simulink library "halin"  (R2021b)
settings: Solver=VariableStepAuto  StartTime=0.0  StopTime=10.0  RelTol=1e-3
undefined symbols (not defined in the file): KHAL_CAN1ABM1E2E_flg, KHAL_CAN1EPB1E2E_flg, KHAL_CAN1EPS1E2E_flg, KHAL_CAN1ESC1E2E_flg, KHAL_CAN1ESC5E2E_flg, KHAL_CAN3BMS1E2E_flg, KHAL_CAN3BMS6E2E_flg, KHAL_CAN3CCU1E2E_flg, KHAL_CAN3CCU2E2E_flg, KHAL_CAN3MCUNF1E2E_flg, KHAL_CAN3MCUNR1E2E_flg, KHAL_CAN3Shifter1E2E_flg, KHAL_CAN3Shifter2E2E_flg, KHAL_CAN6FCM2E2E_flg, KHAL_CAN6FCM4E2E_flg, TRUE
libraries: simulink x645, FVT_lib x207, hcu_lib x59
(part 8 of 23)

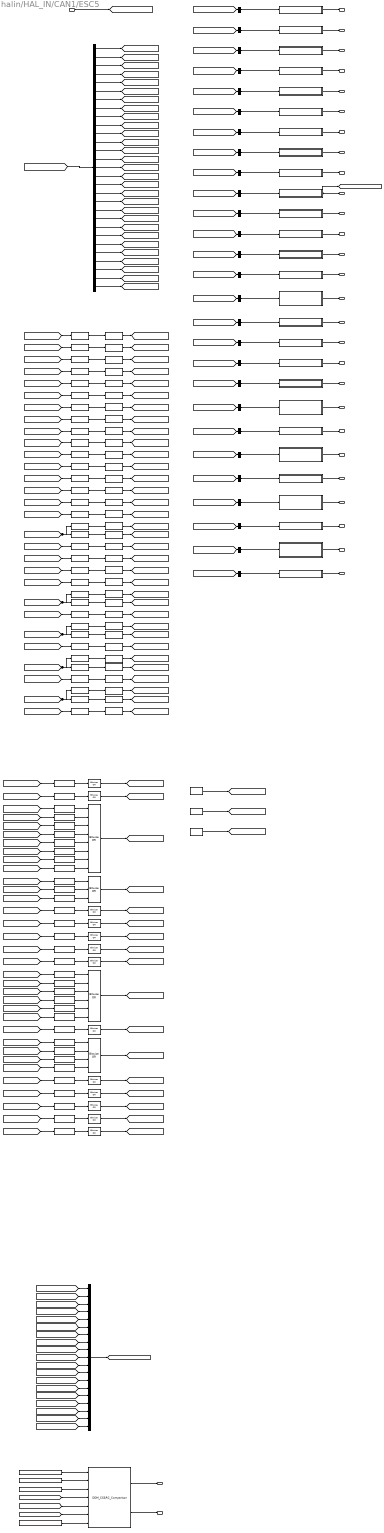
== system halin/HAL_IN/CAN1/ESC5 ==
  DT_CAN1_SG_ESC5 : Inport
  0x59 : Constant  Value=0x59
  0x6E : Constant  Value=0x6E
  ACCAvail : Subsystem
  AEBAvail : Subsystem
  ActBrkLampSta : Subsystem
  BitwiseAND{,1..33} (34 alike) : simulink/Logic and Bit Operations/Bitwise Operator  logicop=AND  UseBitMask=on  BitMask=0xFF  BitMaskRealWorld=Stored Integer
  BitwiseOR{,1,4..8,10,12..16} (13 alike) : simulink/Logic and Bit Operations/Bitwise Operator  logicop=OR  UseBitMask=off  BitMask=bin2dec('11011001')  BitMaskRealWorld=Stored Integer
  BitwiseOR11 : simulink/Logic and Bit Operations/Bitwise Operator  logicop=OR  UseBitMask=off  NumInputPorts=4  BitMask=bin2dec('11011001')  BitMaskRealWorld=Stored Integer
  BitwiseOR2 : simulink/Logic and Bit Operations/Bitwise Operator  logicop=OR  UseBitMask=off  NumInputPorts=8  BitMask=bin2dec('11011001')  BitMaskRealWorld=Stored Integer
  BitwiseOR3 : simulink/Logic and Bit Operations/Bitwise Operator  logicop=OR  UseBitMask=off  NumInputPorts=3  BitMask=bin2dec('11011001')  BitMaskRealWorld=Stored Integer
  BitwiseOR9 : simulink/Logic and Bit Operations/Bitwise Operator  logicop=OR  UseBitMask=off  NumInputPorts=6  BitMask=bin2dec('11011001')  BitMaskRealWorld=Stored Integer
  BrkDiscTempSta : Subsystem
  BrkPedalPos : Subsystem
  BrkPedalPosSta : Subsystem
  BrkSwSta : Subsystem
  BrkSwV : Subsystem
  DDM_CS&RC_Comparison : FVT_lib/hal/DDM_CS&RC_Comparison  MsgCycleTime=10
  Data Type Conversion{,1..33} (34 alike) : DataTypeConversion  OutDataTypeStr=uint8
  ESC5CS : Subsystem
  ESC5RC : Subsystem
  ESCADASSta : Subsystem
  ESCAPSSta : Subsystem
  ESCStandstill : Subsystem
  FrRBCActive : Subsystem
  FrntAxlTrqReqBrk : Subsystem
  KHAL_CAN1ESC5E2E_flg : Constant  Value=KHAL_CAN1ESC5E2E_flg
  LatAccel : Subsystem
  LatAccelV : Subsystem
  LeftShift : ArithShift  BitShiftNumber=1  BitShiftDirection=Left
  LeftShift1 : ArithShift  BitShiftNumber=3  BitShiftDirection=Left
  LeftShift{3..4,9..10,14..16,18} (8 alike) : ArithShift  BitShiftDirection=Left
  LeftShift11 : ArithShift  BitShiftNumber=4  BitShiftDirection=Left
  LeftShift12 : ArithShift  BitShiftNumber=5  BitShiftDirection=Left
  LeftShift13 : ArithShift  BitShiftNumber=7  BitShiftDirection=Left
  LeftShift17 : ArithShift  BitShiftNumber=3  BitShiftDirection=Left
  LeftShift19 : ArithShift  BitShiftNumber=4  BitShiftDirection=Left
  LeftShift2 : ArithShift  BitShiftNumber=2  BitShiftDirection=Left
  LeftShift20 : ArithShift  BitShiftNumber=5  BitShiftDirection=Left
  LeftShift21 : ArithShift  BitShiftNumber=2  BitShiftDirection=Left
  LeftShift22 : ArithShift  BitShiftNumber=1  BitShiftDirection=Left
  LeftShift23 : ArithShift  BitShiftNumber=2  BitShiftDirection=Left
  LeftShift5 : ArithShift  BitShiftNumber=4  BitShiftDirection=Left
  LeftShift6 : ArithShift  BitShiftNumber=6  BitShiftDirection=Left
  LeftShift7 : ArithShift  BitShiftNumber=7  BitShiftDirection=Left
  LeftShift8 : ArithShift  BitShiftNumber=1  BitShiftDirection=Left
  LongAccel : Subsystem
  LongAccelV : Subsystem
  MCPressure : Subsystem
  MCPressureV : Subsystem
  MessageRollingCounter : FVT_lib/hal/MessageRollingCounter  CounterMAX=14  task_time_ms=5  msg_time_ms=10
  MeterIndVehSpeed : Subsystem
  Mux : Mux  Inputs=19
  RDCActive : Subsystem
  RearAxlTrqReqBrk : Subsystem
  RightShift{,2,6,8} (4 alike) : ArithShift  BitShiftNumber=8
  RightShift{1,3,7,9} (4 alike) : ArithShift
  RightShift4 : ArithShift  BitShiftNumber=4
  RightShift5 : ArithShift  BitShiftNumber=-4
  RrRBCActive : Subsystem
  YawRate : Subsystem
  YawRateV : Subsystem
  bus_selector : BusSelector  OutputSignals=CAN1_ACCAvail,CAN1_AEBAvail,CAN1_ActBrkLamp_Sta,CAN1_BrkDiscTempSta,CAN1_BrkPedalPos,CAN1_BrkPedalPos_Sta,CAN1_BrkSw_Sta,CAN1_BrkSw_V,CAN1_DecErrSta,CAN1_ESC5_CS,CAN1_ESC5_RC,CAN1_ESC_ADAS_Sta,CAN1_ESC_APS_Sta,CAN1_ESC_DriverBrkOverride,CAN1_ESC_Standstill,CAN1_Fr_RBC_Active,CAN1_FrntAxlTrqReq_Brk,CAN1_LatAccel,CAN1_LatAccel_V,CAN1_LongAccel,CAN1_LongAccel_V,CAN1_MCPressure,CAN1_MCPressure_V,CAN1_Meter_Ind_VehSpeed,CAN1_RDC_Active,CAN1_RearAxlTrqReq_Brk,CAN1_Rr_RBC_Active,CAN1_YawRate,CAN1_YawRate_V
  bus_selector1 : BusSelector  OutputSignals=CAN1_ACCAvail
  bus_selector10 : BusSelector  OutputSignals=CAN1_ESC5_RC
  bus_selector11 : BusSelector  OutputSignals=CAN1_ESC_ADAS_Sta
  bus_selector12 : BusSelector  OutputSignals=CAN1_ESC_APS_Sta
  bus_selector13 : BusSelector  OutputSignals=CAN1_ESC_Standstill
  bus_selector14 : BusSelector  OutputSignals=CAN1_Fr_RBC_Active
  bus_selector15 : BusSelector  OutputSignals=CAN1_FrntAxlTrqReq_Brk
  bus_selector16 : BusSelector  OutputSignals=CAN1_LatAccel
  bus_selector17 : BusSelector  OutputSignals=CAN1_LatAccel_V
  bus_selector18 : BusSelector  OutputSignals=CAN1_LongAccel
  bus_selector19 : BusSelector  OutputSignals=CAN1_LongAccel_V
  bus_selector2 : BusSelector  OutputSignals=CAN1_AEBAvail
  bus_selector20 : BusSelector  OutputSignals=CAN1_MCPressure
  bus_selector21 : BusSelector  OutputSignals=CAN1_MCPressure_V
  bus_selector22 : BusSelector  OutputSignals=CAN1_Meter_Ind_VehSpeed
  bus_selector23 : BusSelector  OutputSignals=CAN1_RDC_Active
  bus_selector24 : BusSelector  OutputSignals=CAN1_RearAxlTrqReq_Brk
  bus_selector25 : BusSelector  OutputSignals=CAN1_Rr_RBC_Active
  bus_selector26 : BusSelector  OutputSignals=CAN1_YawRate
  bus_selector27 : BusSelector  OutputSignals=CAN1_YawRate_V
  bus_selector3 : BusSelector  OutputSignals=CAN1_ActBrkLamp_Sta
  bus_selector4 : BusSelector  OutputSignals=CAN1_BrkDiscTempSta
  bus_selector5 : BusSelector  OutputSignals=CAN1_BrkPedalPos
  bus_selector6 : BusSelector  OutputSignals=CAN1_BrkPedalPos_Sta
  bus_selector7 : BusSelector  OutputSignals=CAN1_BrkSw_Sta
  bus_selector8 : BusSelector  OutputSignals=CAN1_BrkSw_V
  bus_selector9 : BusSelector  OutputSignals=CAN1_ESC5_CS
  constant : Constant  Value=0x0  OutDataTypeStr=uint8
  constant1 : Constant  Value=0x0  OutDataTypeStr=uint8
  constant2 : Constant  Value=0x0  OutDataTypeStr=uint8
  VHAL_ESC5CSErr_flg : Outport
  VHAL_ESC5RCErr_flg : Outport  Port=2
  VHAL_ACCAvail_flg : Outport  Port=3
  VHAL_AEBAvail_flg : Outport  Port=4
  VHAL_ActBrkLampSta_flg : Outport  Port=5
  VHAL_BrkDiscTempSta_flg : Outport  Port=6
  VHAL_BrkPedalPos_pct : Outport  Port=7
  VHAL_BrkPedalPosSta_flg : Outport  Port=8
  VHAL_BrkSwSta_flg : Outport  Port=9
  VHAL_BrkSwV_flg : Outport  Port=10
  VHAL_ESC5CS_enum : Outport  Port=11
  VHAL_ESC5RC_enum : Outport  Port=12
  VHAL_ESCADASSta_enum : Outport  Port=13
  VHAL_ESCAPSSta_enum : Outport  Port=14
  VHAL_ESCStandstill_flg : Outport  Port=15
  VHAL_FrRBCActive_flg : Outport  Port=16
  VHAL_FrntAxlTrqReqBrk_Nm : Outport  Port=17
  VHAL_LatAccel_Gps : Outport  Port=18
  VHAL_LatAccelV_flg : Outport  Port=19
  VHAL_LongAccel_Gps : Outport  Port=20
  VHAL_LongAccelV_flg : Outport  Port=21
  VHAL_MCPressure_bar : Outport  Port=22
  VHAL_MCPressureV_flg : Outport  Port=23
  VHAL_MeterIndVehSpeed_kph : Outport  Port=24
  VHAL_RDCActive_enum : Outport  Port=25
  VHAL_RearAxlTrqReqBrk_Nm : Outport  Port=26
  VHAL_RrRBCActive_flg : Outport  Port=27
  VHAL_YawRate_degps : Outport  Port=28
  VHAL_YawRateV_flg : Outport  Port=29
  wires:
  DT_CAN1_SG_ESC5/1 -> [DT_CAN1_SG_ESC5]
  [DT_CAN1_SG_ESC5] -> bus_selector/1
  bus_selector/1 -> [CAN1_ACCAvail]  "<CAN1_ACCAvail>"
  [CAN1_ACCAvail] -> LeftShift/1
  LeftShift/1 -> BitwiseAND/1
  BitwiseAND/1 -> [Byte_2_CAN1_ACCAvail]
  bus_selector/2 -> [CAN1_AEBAvail]  "<CAN1_AEBAvail>"
  [CAN1_AEBAvail] -> LeftShift1/1
  LeftShift1/1 -> BitwiseAND1/1
  BitwiseAND1/1 -> [Byte_9_CAN1_AEBAvail]
  bus_selector/3 -> [CAN1_ActBrkLamp_Sta]  "<CAN1_ActBrkLamp_Sta>"
  [CAN1_ActBrkLamp_Sta] -> LeftShift2/1
  LeftShift2/1 -> BitwiseAND2/1
  BitwiseAND2/1 -> [Byte_9_CAN1_ActBrkLamp_Sta]
  bus_selector/4 -> [CAN1_BrkDiscTempSta]  "<CAN1_BrkDiscTempSta>"
  [CAN1_BrkDiscTempSta] -> LeftShift3/1
  LeftShift3/1 -> BitwiseAND3/1
  BitwiseAND3/1 -> [Byte_2_CAN1_BrkDiscTempSta]
  bus_selector/5 -> [CAN1_BrkPedalPos]  "<CAN1_BrkPedalPos>"
  [CAN1_BrkPedalPos] -> LeftShift4/1
  LeftShift4/1 -> BitwiseAND4/1
  BitwiseAND4/1 -> [Byte_12_CAN1_BrkPedalPos]
  bus_selector/6 -> [CAN1_BrkPedalPos_Sta]  "<CAN1_BrkPedalPos_Sta>"
  [CAN1_BrkPedalPos_Sta] -> LeftShift5/1
  LeftShift5/1 -> BitwiseAND5/1
  BitwiseAND5/1 -> [Byte_9_CAN1_BrkPedalPos_Sta]
  bus_selector/7 -> [CAN1_BrkSw_Sta]  "<CAN1_BrkSw_Sta>"
  [CAN1_BrkSw_Sta] -> LeftShift6/1
  LeftShift6/1 -> BitwiseAND6/1
  BitwiseAND6/1 -> [Byte_2_CAN1_BrkSw_Sta]
  bus_selector/8 -> [CAN1_BrkSw_V]  "<CAN1_BrkSw_V>"
  [CAN1_BrkSw_V] -> LeftShift7/1
  LeftShift7/1 -> BitwiseAND7/1
  BitwiseAND7/1 -> [Byte_2_CAN1_BrkSw_V]
  bus_selector/9 -> [CAN1_DecErrSta]  "<CAN1_DecErrSta>"
  [CAN1_DecErrSta] -> LeftShift8/1
  LeftShift8/1 -> BitwiseAND8/1
  BitwiseAND8/1 -> [Byte_9_CAN1_DecErrSta]
  bus_selector/10 -> [CAN1_ESC5_CS]  "<CAN1_ESC5_CS>"
  [CAN1_ESC5_CS] -> LeftShift9/1
  LeftShift9/1 -> BitwiseAND9/1
  BitwiseAND9/1 -> [Byte_0_CAN1_ESC5_CS]
  bus_selector/11 -> [CAN1_ESC5_RC]  "<CAN1_ESC5_RC>"
  [CAN1_ESC5_RC] -> LeftShift10/1
  LeftShift10/1 -> BitwiseAND10/1
  BitwiseAND10/1 -> [Byte_1_CAN1_ESC5_RC]
  bus_selector/12 -> [CAN1_ESC_ADAS_Sta]  "<CAN1_ESC_ADAS_Sta>"
  [CAN1_ESC_ADAS_Sta] -> LeftShift11/1
  LeftShift11/1 -> BitwiseAND11/1
  BitwiseAND11/1 -> [Byte_3_CAN1_ESC_ADAS_Sta]
  bus_selector/13 -> [CAN1_ESC_APS_Sta]  "<CAN1_ESC_APS_Sta>"
  [CAN1_ESC_APS_Sta] -> LeftShift12/1
  LeftShift12/1 -> BitwiseAND12/1
  BitwiseAND12/1 -> [Byte_9_CAN1_ESC_APS_Sta]
  bus_selector/14 -> [CAN1_ESC_DriverBrkOverride]  "<CAN1_ESC_DriverBrkOverride>"
  [CAN1_ESC_DriverBrkOverride] -> LeftShift13/1
  LeftShift13/1 -> BitwiseAND13/1
  BitwiseAND13/1 -> [Byte_3_CAN1_ESC_DriverBrkOverride]
  bus_selector/15 -> [CAN1_ESC_Standstill]  "<CAN1_ESC_Standstill>"
  [CAN1_ESC_Standstill] -> LeftShift14/1
  LeftShift14/1 -> BitwiseAND14/1
  BitwiseAND14/1 -> [Byte_9_CAN1_ESC_Standstill]
  bus_selector/16 -> [CAN1_Fr_RBC_Active]  "<CAN1_Fr_RBC_Active>"
  [CAN1_Fr_RBC_Active] -> LeftShift15/1
  LeftShift15/1 -> BitwiseAND15/1
  BitwiseAND15/1 -> [Byte_11_CAN1_Fr_RBC_Active]
  bus_selector/17 -> [CAN1_FrntAxlTrqReq_Brk]  "<CAN1_FrntAxlTrqReq_Brk>"
  [CAN1_FrntAxlTrqReq_Brk] -> RightShift/1, RightShift1/1
  RightShift/1 -> BitwiseAND16/1
  BitwiseAND16/1 -> [Byte_15_CAN1_FrntAxlTrqReq_Brk]
  RightShift1/1 -> BitwiseAND17/1
  BitwiseAND17/1 -> [Byte_16_CAN1_FrntAxlTrqReq_Brk]
  bus_selector/18 -> [CAN1_LatAccel]  "<CAN1_LatAccel>"
  [CAN1_LatAccel] -> LeftShift16/1
  LeftShift16/1 -> BitwiseAND18/1
  BitwiseAND18/1 -> [Byte_6_CAN1_LatAccel]
  bus_selector/19 -> [CAN1_LatAccel_V]  "<CAN1_LatAccel_V>"
  [CAN1_LatAccel_V] -> LeftShift17/1
  LeftShift17/1 -> BitwiseAND19/1
  BitwiseAND19/1 -> [Byte_2_CAN1_LatAccel_V]
  bus_selector/20 -> [CAN1_LongAccel]  "<CAN1_LongAccel>"
  [CAN1_LongAccel] -> LeftShift18/1
  LeftShift18/1 -> BitwiseAND20/1
  BitwiseAND20/1 -> [Byte_5_CAN1_LongAccel]
  bus_selector/21 -> [CAN1_LongAccel_V]  "<CAN1_LongAccel_V>"
  [CAN1_LongAccel_V] -> LeftShift19/1
  LeftShift19/1 -> BitwiseAND21/1
  BitwiseAND21/1 -> [Byte_2_CAN1_LongAccel_V]
  bus_selector/22 -> [CAN1_MCPressure]  "<CAN1_MCPressure>"
  [CAN1_MCPressure] -> RightShift2/1, RightShift3/1
  RightShift2/1 -> BitwiseAND22/1
  BitwiseAND22/1 -> [Byte_3_CAN1_MCPressure]
  RightShift3/1 -> BitwiseAND23/1
  BitwiseAND23/1 -> [Byte_4_CAN1_MCPressure]
  bus_selector/23 -> [CAN1_MCPressure_V]  "<CAN1_MCPressure_V>"
  [CAN1_MCPressure_V] -> LeftShift20/1
  LeftShift20/1 -> BitwiseAND24/1
  BitwiseAND24/1 -> [Byte_2_CAN1_MCPressure_V]
  bus_selector/24 -> [CAN1_Meter_Ind_VehSpeed]  "<CAN1_Meter_Ind_VehSpeed>"
  [CAN1_Meter_Ind_VehSpeed] -> RightShift4/1, RightShift5/1
  RightShift4/1 -> BitwiseAND25/1
  BitwiseAND25/1 -> [Byte_10_CAN1_Meter_Ind_VehSpeed]
  RightShift5/1 -> BitwiseAND26/1
  BitwiseAND26/1 -> [Byte_11_CAN1_Meter_Ind_VehSpeed]
  bus_selector/25 -> [CAN1_RDC_Active]  "<CAN1_RDC_Active>"
  [CAN1_RDC_Active] -> LeftShift21/1
  LeftShift21/1 -> BitwiseAND27/1
  BitwiseAND27/1 -> [Byte_11_CAN1_RDC_Active]
  bus_selector/26 -> [CAN1_RearAxlTrqReq_Brk]  "<CAN1_RearAxlTrqReq_Brk>"
  [CAN1_RearAxlTrqReq_Brk] -> RightShift6/1, RightShift7/1
  RightShift6/1 -> BitwiseAND28/1
  BitwiseAND28/1 -> [Byte_13_CAN1_RearAxlTrqReq_Brk]
  RightShift7/1 -> BitwiseAND29/1
  BitwiseAND29/1 -> [Byte_14_CAN1_RearAxlTrqReq_Brk]
  bus_selector/27 -> [CAN1_Rr_RBC_Active]  "<CAN1_Rr_RBC_Active>"
  [CAN1_Rr_RBC_Active] -> LeftShift22/1
  LeftShift22/1 -> BitwiseAND30/1
  BitwiseAND30/1 -> [Byte_11_CAN1_Rr_RBC_Active]
  bus_selector/28 -> [CAN1_YawRate]  "<CAN1_YawRate>"
  [CAN1_YawRate] -> RightShift8/1, RightShift9/1
  RightShift8/1 -> BitwiseAND31/1
  BitwiseAND31/1 -> [Byte_7_CAN1_YawRate]
  RightShift9/1 -> BitwiseAND32/1
  BitwiseAND32/1 -> [Byte_8_CAN1_YawRate]
  bus_selector/29 -> [CAN1_YawRate_V]  "<CAN1_YawRate_V>"
  [CAN1_YawRate_V] -> LeftShift23/1
  LeftShift23/1 -> BitwiseAND33/1
  BitwiseAND33/1 -> [Byte_2_CAN1_YawRate_V]
  Data Type Conversion/1 -> BitwiseOR/1
  [Byte_0_CAN1_ESC5_CS] -> Data Type Conversion/1
  BitwiseOR/1 -> [Byte_0]
  Data Type Conversion1/1 -> BitwiseOR1/1
  [Byte_1_CAN1_ESC5_RC] -> Data Type Conversion1/1
  BitwiseOR1/1 -> [Byte_1]
  Data Type Conversion2/1 -> BitwiseOR2/1
  [Byte_2_CAN1_ACCAvail] -> Data Type Conversion2/1
  Data Type Conversion3/1 -> BitwiseOR2/2
  [Byte_2_CAN1_BrkDiscTempSta] -> Data Type Conversion3/1
  Data Type Conversion4/1 -> BitwiseOR2/3
  [Byte_2_CAN1_BrkSw_Sta] -> Data Type Conversion4/1
  Data Type Conversion5/1 -> BitwiseOR2/4
  [Byte_2_CAN1_BrkSw_V] -> Data Type Conversion5/1
  Data Type Conversion6/1 -> BitwiseOR2/5
  [Byte_2_CAN1_LatAccel_V] -> Data Type Conversion6/1
  Data Type Conversion7/1 -> BitwiseOR2/6
  [Byte_2_CAN1_LongAccel_V] -> Data Type Conversion7/1
  Data Type Conversion8/1 -> BitwiseOR2/7
  [Byte_2_CAN1_MCPressure_V] -> Data Type Conversion8/1
  Data Type Conversion9/1 -> BitwiseOR2/8
  [Byte_2_CAN1_YawRate_V] -> Data Type Conversion9/1
  BitwiseOR2/1 -> [Byte_2]
  Data Type Conversion10/1 -> BitwiseOR3/1
  [Byte_3_CAN1_ESC_ADAS_Sta] -> Data Type Conversion10/1
  Data Type Conversion11/1 -> BitwiseOR3/2
  [Byte_3_CAN1_ESC_DriverBrkOverride] -> Data Type Conversion11/1
  Data Type Conversion12/1 -> BitwiseOR3/3
  [Byte_3_CAN1_MCPressure] -> Data Type Conversion12/1
  BitwiseOR3/1 -> [Byte_3]
  Data Type Conversion13/1 -> BitwiseOR4/1
  [Byte_4_CAN1_MCPressure] -> Data Type Conversion13/1
  BitwiseOR4/1 -> [Byte_4]
  Data Type Conversion14/1 -> BitwiseOR5/1
  [Byte_5_CAN1_LongAccel] -> Data Type Conversion14/1
  BitwiseOR5/1 -> [Byte_5]
  Data Type Conversion15/1 -> BitwiseOR6/1
  [Byte_6_CAN1_LatAccel] -> Data Type Conversion15/1
  BitwiseOR6/1 -> [Byte_6]
  Data Type Conversion16/1 -> BitwiseOR7/1
  [Byte_7_CAN1_YawRate] -> Data Type Conversion16/1
  BitwiseOR7/1 -> [Byte_7]
  Data Type Conversion17/1 -> BitwiseOR8/1
  [Byte_8_CAN1_YawRate] -> Data Type Conversion17/1
  BitwiseOR8/1 -> [Byte_8]
  Data Type Conversion18/1 -> BitwiseOR9/1
  [Byte_9_CAN1_AEBAvail] -> Data Type Conversion18/1
  Data Type Conversion19/1 -> BitwiseOR9/2
  [Byte_9_CAN1_ActBrkLamp_Sta] -> Data Type Conversion19/1
  Data Type Conversion20/1 -> BitwiseOR9/3
  [Byte_9_CAN1_BrkPedalPos_Sta] -> Data Type Conversion20/1
  Data Type Conversion21/1 -> BitwiseOR9/4
  [Byte_9_CAN1_DecErrSta] -> Data Type Conversion21/1
  Data Type Conversion22/1 -> BitwiseOR9/5
  [Byte_9_CAN1_ESC_APS_Sta] -> Data Type Conversion22/1
  Data Type Conversion23/1 -> BitwiseOR9/6
  [Byte_9_CAN1_ESC_Standstill] -> Data Type Conversion23/1
  BitwiseOR9/1 -> [Byte_9]
  Data Type Conversion24/1 -> BitwiseOR10/1
  [Byte_10_CAN1_Meter_Ind_VehSpeed] -> Data Type Conversion24/1
  BitwiseOR10/1 -> [Byte_10]
  Data Type Conversion25/1 -> BitwiseOR11/1
  [Byte_11_CAN1_Fr_RBC_Active] -> Data Type Conversion25/1
  Data Type Conversion26/1 -> BitwiseOR11/2
  [Byte_11_CAN1_Meter_Ind_VehSpeed] -> Data Type Conversion26/1
  Data Type Conversion27/1 -> BitwiseOR11/3
  [Byte_11_CAN1_RDC_Active] -> Data Type Conversion27/1
  Data Type Conversion28/1 -> BitwiseOR11/4
  [Byte_11_CAN1_Rr_RBC_Active] -> Data Type Conversion28/1
  BitwiseOR11/1 -> [Byte_11]
  Data Type Conversion29/1 -> BitwiseOR12/1
  [Byte_12_CAN1_BrkPedalPos] -> Data Type Conversion29/1
  BitwiseOR12/1 -> [Byte_12]
  Data Type Conversion30/1 -> BitwiseOR13/1
  [Byte_13_CAN1_RearAxlTrqReq_Brk] -> Data Type Conversion30/1
  BitwiseOR13/1 -> [Byte_13]
  Data Type Conversion31/1 -> BitwiseOR14/1
  [Byte_14_CAN1_RearAxlTrqReq_Brk] -> Data Type Conversion31/1
  BitwiseOR14/1 -> [Byte_14]
  Data Type Conversion32/1 -> BitwiseOR15/1
  [Byte_15_CAN1_FrntAxlTrqReq_Brk] -> Data Type Conversion32/1
  BitwiseOR15/1 -> [Byte_15]
  Data Type Conversion33/1 -> BitwiseOR16/1
  [Byte_16_CAN1_FrntAxlTrqReq_Brk] -> Data Type Conversion33/1
  BitwiseOR16/1 -> [Byte_16]
  constant/1 -> [Byte_17]
  constant1/1 -> [Byte_18]
  constant2/1 -> [Byte_19]
  [Byte_1] -> Mux/1
  [Byte_2] -> Mux/2
  [Byte_3] -> Mux/3
  [Byte_4] -> Mux/4
  [Byte_5] -> Mux/5
  [Byte_6] -> Mux/6
  [Byte_7] -> Mux/7
  [Byte_8] -> Mux/8
  [Byte_9] -> Mux/9
  [Byte_10] -> Mux/10
  [Byte_11] -> Mux/11
  [Byte_12] -> Mux/12
  [Byte_13] -> Mux/13
  [Byte_14] -> Mux/14
  [Byte_15] -> Mux/15
  [Byte_16] -> Mux/16
  [Byte_17] -> Mux/17
  [Byte_18] -> Mux/18
  [Byte_19] -> Mux/19
  Mux/1 -> [VHAL_CAN1ESC5noCS_raw]
  KHAL_CAN1ESC5E2E_flg/1 -> DDM_CS&RC_Comparison/1
  0x59/1 -> DDM_CS&RC_Comparison/2
  0x6E/1 -> DDM_CS&RC_Comparison/3
  [VHAL_CAN1ESC5noCS_raw] -> DDM_CS&RC_Comparison/4
  [Byte_0] -> DDM_CS&RC_Comparison/5
  [RC_ECU] -> DDM_CS&RC_Comparison/6
  MessageRollingCounter/1 -> DDM_CS&RC_Comparison/7
  DDM_CS&RC_Comparison/1 -> VHAL_ESC5CSErr_flg/1
  DDM_CS&RC_Comparison/2 -> VHAL_ESC5RCErr_flg/1
  [DT_CAN1_SG_ESC5] -> bus_selector1/1
  bus_selector1/1 -> ACCAvail/1(ACCAvail)  "<CAN1_ACCAvail>"
  ACCAvail/1(VHAL_ACCAvail_flg) -> VHAL_ACCAvail_flg/1
  [DT_CAN1_SG_ESC5] -> bus_selector2/1
  bus_selector2/1 -> AEBAvail/1(AEBAvail)  "<CAN1_AEBAvail>"
  AEBAvail/1(VHAL_AEBAvail_flg) -> VHAL_AEBAvail_flg/1
  [DT_CAN1_SG_ESC5] -> bus_selector3/1
  bus_selector3/1 -> ActBrkLampSta/1(ActBrkLamp_Sta)  "<CAN1_ActBrkLamp_Sta>"
  ActBrkLampSta/1(VHAL_ActBrkLampSta_flg) -> VHAL_ActBrkLampSta_flg/1
  [DT_CAN1_SG_ESC5] -> bus_selector4/1
  bus_selector4/1 -> BrkDiscTempSta/1(BrkDiscTempSta)  "<CAN1_BrkDiscTempSta>"
  BrkDiscTempSta/1(VHAL_BrkDiscTempSta_flg) -> VHAL_BrkDiscTempSta_flg/1
  [DT_CAN1_SG_ESC5] -> bus_selector5/1
  bus_selector5/1 -> BrkPedalPos/1(BrkPedalPos)  "<CAN1_BrkPedalPos>"
  BrkPedalPos/1(VHAL_BrkPedalPos_pct) -> VHAL_BrkPedalPos_pct/1
  [DT_CAN1_SG_ESC5] -> bus_selector6/1
  bus_selector6/1 -> BrkPedalPosSta/1(BrkPedalPos_Sta)  "<CAN1_BrkPedalPos_Sta>"
  BrkPedalPosSta/1(VHAL_BrkPedalPosSta_flg) -> VHAL_BrkPedalPosSta_flg/1
  [DT_CAN1_SG_ESC5] -> bus_selector7/1
  bus_selector7/1 -> BrkSwSta/1(BrkSw_Sta)  "<CAN1_BrkSw_Sta>"
  BrkSwSta/1(VHAL_BrkSwSta_flg) -> VHAL_BrkSwSta_flg/1
  [DT_CAN1_SG_ESC5] -> bus_selector8/1
  bus_selector8/1 -> BrkSwV/1(BrkSw_V)  "<CAN1_BrkSw_V>"
  BrkSwV/1(VHAL_BrkSwV_flg) -> VHAL_BrkSwV_flg/1
  [DT_CAN1_SG_ESC5] -> bus_selector9/1
  bus_selector9/1 -> ESC5CS/1(ESC5_CS)  "<CAN1_ESC5_CS>"
  ESC5CS/1(VHAL_ESC5CS_enum) -> VHAL_ESC5CS_enum/1
  [DT_CAN1_SG_ESC5] -> bus_selector10/1
  bus_selector10/1 -> ESC5RC/1(ESC5_RC)  "<CAN1_ESC5_RC>"
  ESC5RC/1(VHAL_ESC5RC_enum) -> VHAL_ESC5RC_enum/1, [RC_ECU]
  [DT_CAN1_SG_ESC5] -> bus_selector11/1
  bus_selector11/1 -> ESCADASSta/1(ESC_ADAS_Sta)  "<CAN1_ESC_ADAS_Sta>"
  ESCADASSta/1(VHAL_ESCADASSta_enum) -> VHAL_ESCADASSta_enum/1
  [DT_CAN1_SG_ESC5] -> bus_selector12/1
  bus_selector12/1 -> ESCAPSSta/1(ESC_APS_Sta)  "<CAN1_ESC_APS_Sta>"
  ESCAPSSta/1(VHAL_ESCAPSSta_enum) -> VHAL_ESCAPSSta_enum/1
  [DT_CAN1_SG_ESC5] -> bus_selector13/1
  bus_selector13/1 -> ESCStandstill/1(ESC_Standstill)  "<CAN1_ESC_Standstill>"
  ESCStandstill/1(VHAL_ESCStandstill_flg) -> VHAL_ESCStandstill_flg/1
  [DT_CAN1_SG_ESC5] -> bus_selector14/1
  bus_selector14/1 -> FrRBCActive/1(Fr_RBC_Active)  "<CAN1_Fr_RBC_Active>"
  FrRBCActive/1(VHAL_FrRBCActive_flg) -> VHAL_FrRBCActive_flg/1
  [DT_CAN1_SG_ESC5] -> bus_selector15/1
  bus_selector15/1 -> FrntAxlTrqReqBrk/1(FrntAxlTrqReq_Brk)  "<CAN1_FrntAxlTrqReq_Brk>"
  FrntAxlTrqReqBrk/1(VHAL_FrntAxlTrqReqBrk_Nm) -> VHAL_FrntAxlTrqReqBrk_Nm/1
  [DT_CAN1_SG_ESC5] -> bus_selector16/1
  bus_selector16/1 -> LatAccel/1(LatAccel)  "<CAN1_LatAccel>"
  LatAccel/1(VHAL_LatAccel_Gps) -> VHAL_LatAccel_Gps/1
  [DT_CAN1_SG_ESC5] -> bus_selector17/1
  bus_selector17/1 -> LatAccelV/1(LatAccel_V)  "<CAN1_LatAccel_V>"
  LatAccelV/1(VHAL_LatAccelV_flg) -> VHAL_LatAccelV_flg/1
  [DT_CAN1_SG_ESC5] -> bus_selector18/1
  bus_selector18/1 -> LongAccel/1(LongAccel)  "<CAN1_LongAccel>"
  LongAccel/1(VHAL_LongAccel_Gps) -> VHAL_LongAccel_Gps/1
  [DT_CAN1_SG_ESC5] -> bus_selector19/1
  bus_selector19/1 -> LongAccelV/1(LongAccel_V)  "<CAN1_LongAccel_V>"
  LongAccelV/1(VHAL_LongAccelV_flg) -> VHAL_LongAccelV_flg/1
  [DT_CAN1_SG_ESC5] -> bus_selector20/1
  bus_selector20/1 -> MCPressure/1(MCPressure)  "<CAN1_MCPressure>"
  MCPressure/1(VHAL_MCPressure_bar) -> VHAL_MCPressure_bar/1
  [DT_CAN1_SG_ESC5] -> bus_selector21/1
  bus_selector21/1 -> MCPressureV/1(MCPressure_V)  "<CAN1_MCPressure_V>"
  MCPressureV/1(VHAL_MCPressureV_flg) -> VHAL_MCPressureV_flg/1
  [DT_CAN1_SG_ESC5] -> bus_selector22/1
  bus_selector22/1 -> MeterIndVehSpeed/1(Meter_Ind_VehSpeed)  "<CAN1_Meter_Ind_VehSpeed>"
  MeterIndVehSpeed/1(VHAL_MeterIndVehSpeed_kph) -> VHAL_MeterIndVehSpeed_kph/1
  [DT_CAN1_SG_ESC5] -> bus_selector23/1
  bus_selector23/1 -> RDCActive/1(RDC_Active)  "<CAN1_RDC_Active>"
  RDCActive/1(VHAL_RDCActive_enum) -> VHAL_RDCActive_enum/1
  [DT_CAN1_SG_ESC5] -> bus_selector24/1
  bus_selector24/1 -> RearAxlTrqReqBrk/1(RearAxlTrqReq_Brk)  "<CAN1_RearAxlTrqReq_Brk>"
  RearAxlTrqReqBrk/1(VHAL_RearAxlTrqReqBrk_Nm) -> VHAL_RearAxlTrqReqBrk_Nm/1
  [DT_CAN1_SG_ESC5] -> bus_selector25/1
  bus_selector25/1 -> RrRBCActive/1(Rr_RBC_Active)  "<CAN1_Rr_RBC_Active>"
  RrRBCActive/1(VHAL_RrRBCActive_flg) -> VHAL_RrRBCActive_flg/1
  [DT_CAN1_SG_ESC5] -> bus_selector26/1
  bus_selector26/1 -> YawRate/1(YawRate)  "<CAN1_YawRate>"
  YawRate/1(VHAL_YawRate_degps) -> VHAL_YawRate_degps/1
  [DT_CAN1_SG_ESC5] -> bus_selector27/1
  bus_selector27/1 -> YawRateV/1(YawRate_V)  "<CAN1_YawRate_V>"
  YawRateV/1(VHAL_YawRateV_flg) -> VHAL_YawRateV_flg/1

== system halin/HAL_IN/CAN1/VHAL_CANMsgInvalidABM1_flg ==
  Cast To Boolean13 : DataTypeConversion  OutDataTypeStr=boolean
  Constant : Constant  Value=TRUE
  Latch13 : hcu_lib/Basic_Blocks/Latch
  Switch13 : Switch  Criteria=u2 ~= 0
  Unit Delay : UnitDelay  SampleTime=-1  HasFrameUpgradeWarning=on
  UnitConverter : DataTypeConversion  OutDataTypeStr=boolean
  Out : Outport
  wires:
  Constant/1 -> Switch13/3
  Unit Delay/1 -> Cast To Boolean13/1
  Cast To Boolean13/1 -> Switch13/1, Latch13/1
  Switch13/1 -> UnitConverter/1
  Latch13/1 -> Switch13/2
  UnitConverter/1 -> Unit Delay/1, Out/1  "VHAL_CANMsgInvalidABM1_flg"

== system halin/HAL_IN/CAN1/VHAL_CANMsgInvalidEPB1_flg ==
  Cast To Boolean13 : DataTypeConversion  OutDataTypeStr=boolean
  Constant : Constant  Value=TRUE
  Latch13 : hcu_lib/Basic_Blocks/Latch
  Switch13 : Switch  Criteria=u2 ~= 0
  Unit Delay : UnitDelay  SampleTime=-1  HasFrameUpgradeWarning=on
  UnitConverter : DataTypeConversion  OutDataTypeStr=boolean
  Out : Outport
  wires:
  Constant/1 -> Switch13/3
  Unit Delay/1 -> Cast To Boolean13/1
  Cast To Boolean13/1 -> Switch13/1, Latch13/1
  Switch13/1 -> UnitConverter/1
  Latch13/1 -> Switch13/2
  UnitConverter/1 -> Unit Delay/1, Out/1  "VHAL_CANMsgInvalidEPB1_flg"

== system halin/HAL_IN/CAN1/VHAL_CANMsgInvalidEPS1_flg ==
  Cast To Boolean13 : DataTypeConversion  OutDataTypeStr=boolean
  Constant : Constant  Value=TRUE
  Latch13 : hcu_lib/Basic_Blocks/Latch
  Switch13 : Switch  Criteria=u2 ~= 0
  Unit Delay : UnitDelay  SampleTime=-1  HasFrameUpgradeWarning=on
  UnitConverter : DataTypeConversion  OutDataTypeStr=boolean
  Out : Outport
  wires:
  Constant/1 -> Switch13/3
  Unit Delay/1 -> Cast To Boolean13/1
  Cast To Boolean13/1 -> Switch13/1, Latch13/1
  Switch13/1 -> UnitConverter/1
  Latch13/1 -> Switch13/2
  UnitConverter/1 -> Unit Delay/1, Out/1  "VHAL_CANMsgInvalidEPS1_flg"

== system halin/HAL_IN/CAN1/VHAL_CANMsgInvalidESC1_flg ==
  Cast To Boolean13 : DataTypeConversion  OutDataTypeStr=boolean
  Constant : Constant  Value=TRUE
  Latch13 : hcu_lib/Basic_Blocks/Latch
  Switch13 : Switch  Criteria=u2 ~= 0
  Unit Delay : UnitDelay  SampleTime=-1  HasFrameUpgradeWarning=on
  UnitConverter : DataTypeConversion  OutDataTypeStr=boolean
  Out : Outport
  wires:
  Constant/1 -> Switch13/3
  Unit Delay/1 -> Cast To Boolean13/1
  Cast To Boolean13/1 -> Switch13/1, Latch13/1
  Switch13/1 -> UnitConverter/1
  Latch13/1 -> Switch13/2
  UnitConverter/1 -> Unit Delay/1, Out/1  "VHAL_CANMsgInvalidESC1_flg"

== system halin/HAL_IN/CAN1/VHAL_CANMsgInvalidESC5_flg ==
  Cast To Boolean13 : DataTypeConversion  OutDataTypeStr=boolean
  Constant : Constant  Value=TRUE
  Latch13 : hcu_lib/Basic_Blocks/Latch
  Switch13 : Switch  Criteria=u2 ~= 0
  Unit Delay : UnitDelay  SampleTime=-1  HasFrameUpgradeWarning=on
  UnitConverter : DataTypeConversion  OutDataTypeStr=boolean
  Out : Outport
  wires:
  Constant/1 -> Switch13/3
  Unit Delay/1 -> Cast To Boolean13/1
  Cast To Boolean13/1 -> Switch13/1, Latch13/1
  Switch13/1 -> UnitConverter/1
  Latch13/1 -> Switch13/2
  UnitConverter/1 -> Unit Delay/1, Out/1  "VHAL_CANMsgInvalidESC5_flg"

== system halin/HAL_IN/CAN1/VHAL_CANMsgInvalideBST1_flg ==
  Cast To Boolean13 : DataTypeConversion  OutDataTypeStr=boolean
  Constant : Constant  Value=TRUE
  Latch13 : hcu_lib/Basic_Blocks/Latch
  Switch13 : Switch  Criteria=u2 ~= 0
  Unit Delay : UnitDelay  SampleTime=-1  HasFrameUpgradeWarning=on
  UnitConverter : DataTypeConversion  OutDataTypeStr=boolean
  Out : Outport
  wires:
  Constant/1 -> Switch13/3
  Unit Delay/1 -> Cast To Boolean13/1
  Cast To Boolean13/1 -> Switch13/1, Latch13/1
  Switch13/1 -> UnitConverter/1
  Latch13/1 -> Switch13/2
  UnitConverter/1 -> Unit Delay/1, Out/1  "VHAL_CANMsgInvalideBST1_flg"

== system halin/HAL_IN/CAN1/eBST1 ==
  DT_CAN1_SG_eBST1 : Inport
  LowBrakeFluidSta : Subsystem
  bus_selector : BusSelector  OutputSignals=CAN1_LowBrakeFluid_Sta
  bus_selector1 : BusSelector  OutputSignals=CAN1_eBST_AmberWnlmpSta
  bus_selector2 : BusSelector  OutputSignals=CAN1_eBST_BeepReq
  bus_selector3 : BusSelector  OutputSignals=CAN1_eBST_RedWnlmpSta
  eBSTAmberWnlmpSta : Subsystem
  eBSTBeepReq : Subsystem
  eBSTRedWnlmpSta : Subsystem
  VHAL_LowBrakeFluidSta_flg : Outport
  VHAL_eBSTAmberWnlmpSta_flg : Outport  Port=2
  VHAL_eBSTBeepReq_flg : Outport  Port=3
  VHAL_eBSTRedWnlmpSta_flg : Outport  Port=4
  wires:
  DT_CAN1_SG_eBST1/1 -> [DT_CAN1_SG_eBST1]
  [DT_CAN1_SG_eBST1] -> bus_selector/1
  bus_selector/1 -> LowBrakeFluidSta/1(LowBrakeFluid_Sta)  "<CAN1_LowBrakeFluid_Sta>"
  LowBrakeFluidSta/1(VHAL_LowBrakeFluidSta_flg) -> VHAL_LowBrakeFluidSta_flg/1
  [DT_CAN1_SG_eBST1] -> bus_selector1/1
  bus_selector1/1 -> eBSTAmberWnlmpSta/1(eBST_AmberWnlmpSta)  "<CAN1_eBST_AmberWnlmpSta>"
  eBSTAmberWnlmpSta/1(VHAL_eBSTAmberWnlmpSta_flg) -> VHAL_eBSTAmberWnlmpSta_flg/1
  [DT_CAN1_SG_eBST1] -> bus_selector2/1
  bus_selector2/1 -> eBSTBeepReq/1(eBST_BeepReq)  "<CAN1_eBST_BeepReq>"
  eBSTBeepReq/1(VHAL_eBSTBeepReq_flg) -> VHAL_eBSTBeepReq_flg/1
  [DT_CAN1_SG_eBST1] -> bus_selector3/1
  bus_selector3/1 -> eBSTRedWnlmpSta/1(eBST_RedWnlmpSta)  "<CAN1_eBST_RedWnlmpSta>"
  eBSTRedWnlmpSta/1(VHAL_eBSTRedWnlmpSta_flg) -> VHAL_eBSTRedWnlmpSta_flg/1

== system halin/HAL_IN/CAN2/HMI1 ==
  DT_CAN2_SG_HMI1 : Inport
  HMIACAirIntMCmd : Subsystem
  HMIACAirIntPCmd : Subsystem
  HMIACAutoBtnCmd : Subsystem
  HMIACBtnCmd : Subsystem
  HMIACFrDefogBtnCmd : Subsystem
  HMIACRecycleBtnCmd : Subsystem
  HMIACWindDirMCmd : Subsystem
  HMIACWindDirPCmd : Subsystem
  HMIAutoInterLightCmd : Subsystem
  HMIBCMPostDefogBtnCmd : Subsystem
  HMIZ1SetTMCmd : Subsystem
  HMIZ1SetTPCmd : Subsystem
  HMIZ2SetTMCmd : Subsystem
  HMIZ2SetTPCmd : Subsystem
  bus_selector : BusSelector  OutputSignals=CAN2_HMI_ACAirIntM_Cmd
  bus_selector1 : BusSelector  OutputSignals=CAN2_HMI_ACAirIntP_Cmd
  bus_selector10 : BusSelector  OutputSignals=CAN2_HMI_Z1SetTM_Cmd
  bus_selector11 : BusSelector  OutputSignals=CAN2_HMI_Z1SetTP_Cmd
  bus_selector12 : BusSelector  OutputSignals=CAN2_HMI_Z2SetTM_Cmd
  bus_selector13 : BusSelector  OutputSignals=CAN2_HMI_Z2SetTP_Cmd
  bus_selector2 : BusSelector  OutputSignals=CAN2_HMI_ACAutoBtn_Cmd
  bus_selector3 : BusSelector  OutputSignals=CAN2_HMI_ACBtn_Cmd
  bus_selector4 : BusSelector  OutputSignals=CAN2_HMI_ACFrDefogBtn_Cmd
  bus_selector5 : BusSelector  OutputSignals=CAN2_HMI_ACRecycleBtn_Cmd
  bus_selector6 : BusSelector  OutputSignals=CAN2_HMI_ACWindDirM_Cmd
  bus_selector7 : BusSelector  OutputSignals=CAN2_HMI_ACWindDirP_Cmd
  bus_selector8 : BusSelector  OutputSignals=CAN2_HMI_AutoInterLight_Cmd
  bus_selector9 : BusSelector  OutputSignals=CAN2_HMI_BCMPostDefogBtn_Cmd
  VHAL_HMIACAirIntMCmd_flg : Outport
  VHAL_HMIACAirIntPCmd_flg : Outport  Port=2
  VHAL_HMIACAutoBtnCmd_flg : Outport  Port=3
  VHAL_HMIACBtnCmd_flg : Outport  Port=4
  VHAL_HMIACFrDefogBtnCmd_flg : Outport  Port=5
  VHAL_HMIACRecycleBtnCmd_flg : Outport  Port=6
  VHAL_HMIACWindDirMCmd_flg : Outport  Port=7
  VHAL_HMIACWindDirPCmd_flg : Outport  Port=8
  VHAL_HMIAutoInterLightCmd_flg : Outport  Port=9
  VHAL_HMIBCMPostDefogBtnCmd_flg : Outport  Port=10
  VHAL_HMIZ1SetTMCmd_flg : Outport  Port=11
  VHAL_HMIZ1SetTPCmd_flg : Outport  Port=12
  VHAL_HMIZ2SetTMCmd_flg : Outport  Port=13
  VHAL_HMIZ2SetTPCmd_flg : Outport  Port=14
  wires:
  DT_CAN2_SG_HMI1/1 -> [DT_CAN2_SG_HMI1]
  [DT_CAN2_SG_HMI1] -> bus_selector/1
  bus_selector/1 -> HMIACAirIntMCmd/1(HMI_ACAirIntM_Cmd)  "<CAN2_HMI_ACAirIntM_Cmd>"
  HMIACAirIntMCmd/1(VHAL_HMIACAirIntMCmd_flg) -> VHAL_HMIACAirIntMCmd_flg/1
  [DT_CAN2_SG_HMI1] -> bus_selector1/1
  bus_selector1/1 -> HMIACAirIntPCmd/1(HMI_ACAirIntP_Cmd)  "<CAN2_HMI_ACAirIntP_Cmd>"
  HMIACAirIntPCmd/1(VHAL_HMIACAirIntPCmd_flg) -> VHAL_HMIACAirIntPCmd_flg/1
  [DT_CAN2_SG_HMI1] -> bus_selector2/1
  bus_selector2/1 -> HMIACAutoBtnCmd/1(HMI_ACAutoBtn_Cmd)  "<CAN2_HMI_ACAutoBtn_Cmd>"
  HMIACAutoBtnCmd/1(VHAL_HMIACAutoBtnCmd_flg) -> VHAL_HMIACAutoBtnCmd_flg/1
  [DT_CAN2_SG_HMI1] -> bus_selector3/1
  bus_selector3/1 -> HMIACBtnCmd/1(HMI_ACBtn_Cmd)  "<CAN2_HMI_ACBtn_Cmd>"
  HMIACBtnCmd/1(VHAL_HMIACBtnCmd_flg) -> VHAL_HMIACBtnCmd_flg/1
  [DT_CAN2_SG_HMI1] -> bus_selector4/1
  bus_selector4/1 -> HMIACFrDefogBtnCmd/1(HMI_ACFrDefogBtn_Cmd)  "<CAN2_HMI_ACFrDefogBtn_Cmd>"
  HMIACFrDefogBtnCmd/1(VHAL_HMIACFrDefogBtnCmd_flg) -> VHAL_HMIACFrDefogBtnCmd_flg/1
  [DT_CAN2_SG_HMI1] -> bus_selector5/1
  bus_selector5/1 -> HMIACRecycleBtnCmd/1(HMI_ACRecycleBtn_Cmd)  "<CAN2_HMI_ACRecycleBtn_Cmd>"
  HMIACRecycleBtnCmd/1(VHAL_HMIACRecycleBtnCmd_flg) -> VHAL_HMIACRecycleBtnCmd_flg/1
  [DT_CAN2_SG_HMI1] -> bus_selector6/1
  bus_selector6/1 -> HMIACWindDirMCmd/1(HMI_ACWindDirM_Cmd)  "<CAN2_HMI_ACWindDirM_Cmd>"
  HMIACWindDirMCmd/1(VHAL_HMIACWindDirMCmd_flg) -> VHAL_HMIACWindDirMCmd_flg/1
  [DT_CAN2_SG_HMI1] -> bus_selector7/1
  bus_selector7/1 -> HMIACWindDirPCmd/1(HMI_ACWindDirP_Cmd)  "<CAN2_HMI_ACWindDirP_Cmd>"
  HMIACWindDirPCmd/1(VHAL_HMIACWindDirPCmd_flg) -> VHAL_HMIACWindDirPCmd_flg/1
  [DT_CAN2_SG_HMI1] -> bus_selector8/1
  bus_selector8/1 -> HMIAutoInterLightCmd/1(HMI_AutoInterLight_Cmd)  "<CAN2_HMI_AutoInterLight_Cmd>"
  HMIAutoInterLightCmd/1(VHAL_HMIAutoInterLightCmd_flg) -> VHAL_HMIAutoInterLightCmd_flg/1
  [DT_CAN2_SG_HMI1] -> bus_selector9/1
  bus_selector9/1 -> HMIBCMPostDefogBtnCmd/1(HMI_BCMPostDefogBtn_Cmd)  "<CAN2_HMI_BCMPostDefogBtn_Cmd>"
  HMIBCMPostDefogBtnCmd/1(VHAL_HMIBCMPostDefogBtnCmd_flg) -> VHAL_HMIBCMPostDefogBtnCmd_flg/1
  [DT_CAN2_SG_HMI1] -> bus_selector10/1
  bus_selector10/1 -> HMIZ1SetTMCmd/1(HMI_Z1SetTM_Cmd)  "<CAN2_HMI_Z1SetTM_Cmd>"
  HMIZ1SetTMCmd/1(VHAL_HMIZ1SetTMCmd_flg) -> VHAL_HMIZ1SetTMCmd_flg/1
  [DT_CAN2_SG_HMI1] -> bus_selector11/1
  bus_selector11/1 -> HMIZ1SetTPCmd/1(HMI_Z1SetTP_Cmd)  "<CAN2_HMI_Z1SetTP_Cmd>"
  HMIZ1SetTPCmd/1(VHAL_HMIZ1SetTPCmd_flg) -> VHAL_HMIZ1SetTPCmd_flg/1
  [DT_CAN2_SG_HMI1] -> bus_selector12/1
  bus_selector12/1 -> HMIZ2SetTMCmd/1(HMI_Z2SetTM_Cmd)  "<CAN2_HMI_Z2SetTM_Cmd>"
  HMIZ2SetTMCmd/1(VHAL_HMIZ2SetTMCmd_flg) -> VHAL_HMIZ2SetTMCmd_flg/1
  [DT_CAN2_SG_HMI1] -> bus_selector13/1
  bus_selector13/1 -> HMIZ2SetTPCmd/1(HMI_Z2SetTP_Cmd)  "<CAN2_HMI_Z2SetTP_Cmd>"
  HMIZ2SetTPCmd/1(VHAL_HMIZ2SetTPCmd_flg) -> VHAL_HMIZ2SetTPCmd_flg/1

== system halin/HAL_IN/CAN2/IVI1 ==
  DT_CAN2_SG_IVI1 : Inport
  AmbLighLowBatAlertSW : Subsystem
  AmbLighSafetyAlertSW : Subsystem
  AmbLightBrightnessSet : Subsystem
  AmbLightColorSet : Subsystem
  AmbLightDimInDarkSW : Subsystem
  AmbLightSW : Subsystem
  AmbLightWlcmLightSW : Subsystem
  FCPFrEvtBtnACMaxReq : Subsystem
  FCPFrEvtBtnACReq : Subsystem
  FCPFrEvtBtnAutoReq : Subsystem
  FCPFrEvtBtnSyncReq : Subsystem
  IVIAutoWipHSpdSWCmd : Subsystem
  IVICreateAccReqSta : Subsystem
  IVIDelAccReqSta : Subsystem
  IVIDrivingLockSWSta : Subsystem
  IVIFrTrunkUnlockReqSta : Subsystem
  IVILinkAccReqSta : Subsystem
  IVILinkAccSta : Subsystem
  IVILinkKeySta : Subsystem
  IVILocatedSTA : Subsystem
  IVILockSoundSWSta : Subsystem
  IVISWCVibModeSta : Subsystem
  IVIStoppingUnlockSWSta : Subsystem
  IVITimeCheck : Subsystem
  IVITimeDay : Subsystem
  IVITimeHour : Subsystem
  IVITimeMinute : Subsystem
  IVITimeMonth : Subsystem
  IVITimeSecond : Subsystem
  IVITimeYear : Subsystem
  IVIWPTCSWSta : Subsystem
  IVIsigScreenReqSta : Subsystem
  LINKtoDrive : Subsystem
  OpenDrOpenWdoSW : Subsystem
  PWCONTINUEUSE : Subsystem
  SmartEcoModeSW : Subsystem
  UserSet : Subsystem
  bus_selector : BusSelector  OutputSignals=CAN2_AmbLigh_LowBatAlert_SW
  bus_selector1 : BusSelector  OutputSignals=CAN2_AmbLigh_SafetyAlert_SW
  bus_selector10 : BusSelector  OutputSignals=CAN2_FCP_FrEvt_BtnSyncReq
  bus_selector11 : BusSelector  OutputSignals=CAN2_IVI_AutoWipHSpdSW_Cmd
  bus_selector12 : BusSelector  OutputSignals=CAN2_IVI_CreateAccReq_Sta
  bus_selector13 : BusSelector  OutputSignals=CAN2_IVI_DelAccReq_Sta
  bus_selector14 : BusSelector  OutputSignals=CAN2_IVI_Driving_Lock_SW_Sta
  bus_selector15 : BusSelector  OutputSignals=CAN2_IVI_FrTrunk_UnlockReq_Sta
  bus_selector16 : BusSelector  OutputSignals=CAN2_IVI_LinkAccReq_Sta
  bus_selector17 : BusSelector  OutputSignals=CAN2_IVI_LinkAcc_Sta
  bus_selector18 : BusSelector  OutputSignals=CAN2_IVI_LinkKey_Sta
  bus_selector19 : BusSelector  OutputSignals=CAN2_IVI_Located_STA
  bus_selector2 : BusSelector  OutputSignals=CAN2_AmbLightBrightnessSet
  bus_selector20 : BusSelector  OutputSignals=CAN2_IVI_Lock_SoundSW_Sta
  bus_selector21 : BusSelector  OutputSignals=CAN2_IVI_SWC_VibMode_Sta
  bus_selector22 : BusSelector  OutputSignals=CAN2_IVI_Stopping_Unlock_SW_Sta
  bus_selector23 : BusSelector  OutputSignals=CAN2_IVI_Time_Check
  bus_selector24 : BusSelector  OutputSignals=CAN2_IVI_Time_Day
  bus_selector25 : BusSelector  OutputSignals=CAN2_IVI_Time_Hour
  bus_selector26 : BusSelector  OutputSignals=CAN2_IVI_Time_Minute
  bus_selector27 : BusSelector  OutputSignals=CAN2_IVI_Time_Month
  bus_selector28 : BusSelector  OutputSignals=CAN2_IVI_Time_Second
  bus_selector29 : BusSelector  OutputSignals=CAN2_IVI_Time_Year
  bus_selector3 : BusSelector  OutputSignals=CAN2_AmbLightColorSet
  bus_selector30 : BusSelector  OutputSignals=CAN2_IVI_WPTC_SW_Sta
  bus_selector31 : BusSelector  OutputSignals=CAN2_IVI_sigScreenReq_Sta
  bus_selector32 : BusSelector  OutputSignals=CAN2_LINKtoDrive
  bus_selector33 : BusSelector  OutputSignals=CAN2_OpenDrOpenWdo_SW
  bus_selector34 : BusSelector  OutputSignals=CAN2_PW_CONTINUE_USE
  bus_selector35 : BusSelector  OutputSignals=CAN2_SmartEco_Mode_SW
  bus_selector36 : BusSelector  OutputSignals=CAN2_UserSet
  bus_selector4 : BusSelector  OutputSignals=CAN2_AmbLight_DimInDark_SW
  bus_selector5 : BusSelector  OutputSignals=CAN2_AmbLight_SW
  bus_selector6 : BusSelector  OutputSignals=CAN2_AmbLight_WlcmLight_SW
  bus_selector7 : BusSelector  OutputSignals=CAN2_FCP_FrEvt_BtnACMaxReq
  bus_selector8 : BusSelector  OutputSignals=CAN2_FCP_FrEvt_BtnACReq
  bus_selector9 : BusSelector  OutputSignals=CAN2_FCP_FrEvt_BtnAutoReq
  VHAL_AmbLighLowBatAlertSW_flg : Outport
  VHAL_AmbLighSafetyAlertSW_flg : Outport  Port=2
  VHAL_AmbLightBrightnessSet_enum : Outport  Port=3
  VHAL_AmbLightColorSet_enum : Outport  Port=4
  VHAL_AmbLightDimInDarkSW_flg : Outport  Port=5
  VHAL_AmbLightSW_flg : Outport  Port=6
  VHAL_AmbLightWlcmLightSW_flg : Outport  Port=7
  VHAL_FCPFrEvtBtnACMaxReq_flg : Outport  Port=8
  VHAL_FCPFrEvtBtnACReq_flg : Outport  Port=9
  VHAL_FCPFrEvtBtnAutoReq_flg : Outport  Port=10
  VHAL_FCPFrEvtBtnSyncReq_flg : Outport  Port=11
  VHAL_IVIAutoWipHSpdSWCmd_flg : Outport  Port=12
  VHAL_IVICreateAccReqSta_enum : Outport  Port=13
  VHAL_IVIDelAccReqSta_enum : Outport  Port=14
  VHAL_IVIDrivingLockSWSta_flg : Outport  Port=15
  VHAL_IVIFrTrunkUnlockReqSta_flg : Outport  Port=16
  VHAL_IVILinkAccReqSta_flg : Outport  Port=17
  VHAL_IVILinkAccSta_enum : Outport  Port=18
  VHAL_IVILinkKeySta_enum : Outport  Port=19
  VHAL_IVILocatedSTA_enum : Outport  Port=20
  VHAL_IVILockSoundSWSta_flg : Outport  Port=21
  VHAL_IVISWCVibModeSta_enum : Outport  Port=22
  VHAL_IVIStoppingUnlockSWSta_flg : Outport  Port=23
  VHAL_IVITimeCheck_enum : Outport  Port=24
  VHAL_IVITimeDay_DAY : Outport  Port=25
  VHAL_IVITimeHour_hr : Outport  Port=26
  VHAL_IVITimeMinute_min : Outport  Port=27
  VHAL_IVITimeMonth_MONTH : Outport  Port=28
  VHAL_IVITimeSecond_s : Outport  Port=29
  VHAL_IVITimeYear_YEAR : Outport  Port=30
  VHAL_IVIWPTCSWSta_flg : Outport  Port=31
  VHAL_IVIsigScreenReqSta_flg : Outport  Port=32
  VHAL_LINKtoDrive_flg : Outport  Port=33
  VHAL_OpenDrOpenWdoSW_flg : Outport  Port=34
  VHAL_PWCONTINUEUSE_flg : Outport  Port=35
  VHAL_SmartEcoModeSW_flg : Outport  Port=36
  VHAL_UserSet_enum : Outport  Port=37
  wires:
  DT_CAN2_SG_IVI1/1 -> [DT_CAN2_SG_IVI1]
  [DT_CAN2_SG_IVI1] -> bus_selector/1
  bus_selector/1 -> AmbLighLowBatAlertSW/1(AmbLigh_LowBatAlert_SW)  "<CAN2_AmbLigh_LowBatAlert_SW>"
  AmbLighLowBatAlertSW/1(VHAL_AmbLighLowBatAlertSW_flg) -> VHAL_AmbLighLowBatAlertSW_flg/1
  [DT_CAN2_SG_IVI1] -> bus_selector1/1
  bus_selector1/1 -> AmbLighSafetyAlertSW/1(AmbLigh_SafetyAlert_SW)  "<CAN2_AmbLigh_SafetyAlert_SW>"
  AmbLighSafetyAlertSW/1(VHAL_AmbLighSafetyAlertSW_flg) -> VHAL_AmbLighSafetyAlertSW_flg/1
  [DT_CAN2_SG_IVI1] -> bus_selector2/1
  bus_selector2/1 -> AmbLightBrightnessSet/1(AmbLightBrightnessSet)  "<CAN2_AmbLightBrightnessSet>"
  AmbLightBrightnessSet/1(VHAL_AmbLightBrightnessSet_enum) -> VHAL_AmbLightBrightnessSet_enum/1
  [DT_CAN2_SG_IVI1] -> bus_selector3/1
  bus_selector3/1 -> AmbLightColorSet/1(AmbLightColorSet)  "<CAN2_AmbLightColorSet>"
  AmbLightColorSet/1(VHAL_AmbLightColorSet_enum) -> VHAL_AmbLightColorSet_enum/1
  [DT_CAN2_SG_IVI1] -> bus_selector4/1
  bus_selector4/1 -> AmbLightDimInDarkSW/1(AmbLight_DimInDark_SW)  "<CAN2_AmbLight_DimInDark_SW>"
  AmbLightDimInDarkSW/1(VHAL_AmbLightDimInDarkSW_flg) -> VHAL_AmbLightDimInDarkSW_flg/1
  [DT_CAN2_SG_IVI1] -> bus_selector5/1
  bus_selector5/1 -> AmbLightSW/1(AmbLight_SW)  "<CAN2_AmbLight_SW>"
  AmbLightSW/1(VHAL_AmbLightSW_flg) -> VHAL_AmbLightSW_flg/1
  [DT_CAN2_SG_IVI1] -> bus_selector6/1
  bus_selector6/1 -> AmbLightWlcmLightSW/1(AmbLight_WlcmLight_SW)  "<CAN2_AmbLight_WlcmLight_SW>"
  AmbLightWlcmLightSW/1(VHAL_AmbLightWlcmLightSW_flg) -> VHAL_AmbLightWlcmLightSW_flg/1
  [DT_CAN2_SG_IVI1] -> bus_selector7/1
  bus_selector7/1 -> FCPFrEvtBtnACMaxReq/1(FCP_FrEvt_BtnACMaxReq)  "<CAN2_FCP_FrEvt_BtnACMaxReq>"
  FCPFrEvtBtnACMaxReq/1(VHAL_FCPFrEvtBtnACMaxReq_flg) -> VHAL_FCPFrEvtBtnACMaxReq_flg/1
  [DT_CAN2_SG_IVI1] -> bus_selector8/1
  bus_selector8/1 -> FCPFrEvtBtnACReq/1(FCP_FrEvt_BtnACReq)  "<CAN2_FCP_FrEvt_BtnACReq>"
  FCPFrEvtBtnACReq/1(VHAL_FCPFrEvtBtnACReq_flg) -> VHAL_FCPFrEvtBtnACReq_flg/1
  [DT_CAN2_SG_IVI1] -> bus_selector9/1
  bus_selector9/1 -> FCPFrEvtBtnAutoReq/1(FCP_FrEvt_BtnAutoReq)  "<CAN2_FCP_FrEvt_BtnAutoReq>"
  FCPFrEvtBtnAutoReq/1(VHAL_FCPFrEvtBtnAutoReq_flg) -> VHAL_FCPFrEvtBtnAutoReq_flg/1
  [DT_CAN2_SG_IVI1] -> bus_selector10/1
  bus_selector10/1 -> FCPFrEvtBtnSyncReq/1(FCP_FrEvt_BtnSyncReq)  "<CAN2_FCP_FrEvt_BtnSyncReq>"
  FCPFrEvtBtnSyncReq/1(VHAL_FCPFrEvtBtnSyncReq_flg) -> VHAL_FCPFrEvtBtnSyncReq_flg/1
  [DT_CAN2_SG_IVI1] -> bus_selector11/1
  bus_selector11/1 -> IVIAutoWipHSpdSWCmd/1(IVI_AutoWipHSpdSW_Cmd)  "<CAN2_IVI_AutoWipHSpdSW_Cmd>"
  IVIAutoWipHSpdSWCmd/1(VHAL_IVIAutoWipHSpdSWCmd_flg) -> VHAL_IVIAutoWipHSpdSWCmd_flg/1
  [DT_CAN2_SG_IVI1] -> bus_selector12/1
  bus_selector12/1 -> IVICreateAccReqSta/1(IVI_CreateAccReq_Sta)  "<CAN2_IVI_CreateAccReq_Sta>"
  IVICreateAccReqSta/1(VHAL_IVICreateAccReqSta_enum) -> VHAL_IVICreateAccReqSta_enum/1
  [DT_CAN2_SG_IVI1] -> bus_selector13/1
  bus_selector13/1 -> IVIDelAccReqSta/1(IVI_DelAccReq_Sta)  "<CAN2_IVI_DelAccReq_Sta>"
  IVIDelAccReqSta/1(VHAL_IVIDelAccReqSta_enum) -> VHAL_IVIDelAccReqSta_enum/1
  [DT_CAN2_SG_IVI1] -> bus_selector14/1
  bus_selector14/1 -> IVIDrivingLockSWSta/1(IVI_Driving_Lock_SW_Sta)  "<CAN2_IVI_Driving_Lock_SW_Sta>"
  IVIDrivingLockSWSta/1(VHAL_IVIDrivingLockSWSta_flg) -> VHAL_IVIDrivingLockSWSta_flg/1
  [DT_CAN2_SG_IVI1] -> bus_selector15/1
  bus_selector15/1 -> IVIFrTrunkUnlockReqSta/1(IVI_FrTrunk_UnlockReq_Sta)  "<CAN2_IVI_FrTrunk_UnlockReq_Sta>"
  IVIFrTrunkUnlockReqSta/1(VHAL_IVIFrTrunkUnlockReqSta_flg) -> VHAL_IVIFrTrunkUnlockReqSta_flg/1
  [DT_CAN2_SG_IVI1] -> bus_selector16/1
  bus_selector16/1 -> IVILinkAccReqSta/1(IVI_LinkAccReq_Sta)  "<CAN2_IVI_LinkAccReq_Sta>"
  IVILinkAccReqSta/1(VHAL_IVILinkAccReqSta_flg) -> VHAL_IVILinkAccReqSta_flg/1
  [DT_CAN2_SG_IVI1] -> bus_selector17/1
  bus_selector17/1 -> IVILinkAccSta/1(IVI_LinkAcc_Sta)  "<CAN2_IVI_LinkAcc_Sta>"
  IVILinkAccSta/1(VHAL_IVILinkAccSta_enum) -> VHAL_IVILinkAccSta_enum/1
  [DT_CAN2_SG_IVI1] -> bus_selector18/1
  bus_selector18/1 -> IVILinkKeySta/1(IVI_LinkKey_Sta)  "<CAN2_IVI_LinkKey_Sta>"
  IVILinkKeySta/1(VHAL_IVILinkKeySta_enum) -> VHAL_IVILinkKeySta_enum/1
  [DT_CAN2_SG_IVI1] -> bus_selector19/1
  bus_selector19/1 -> IVILocatedSTA/1(IVI_Located_STA)  "<CAN2_IVI_Located_STA>"
  IVILocatedSTA/1(VHAL_IVILocatedSTA_enum) -> VHAL_IVILocatedSTA_enum/1
  [DT_CAN2_SG_IVI1] -> bus_selector20/1
  bus_selector20/1 -> IVILockSoundSWSta/1(IVI_Lock_SoundSW_Sta)  "<CAN2_IVI_Lock_SoundSW_Sta>"
  IVILockSoundSWSta/1(VHAL_IVILockSoundSWSta_flg) -> VHAL_IVILockSoundSWSta_flg/1
  [DT_CAN2_SG_IVI1] -> bus_selector21/1
  bus_selector21/1 -> IVISWCVibModeSta/1(IVI_SWC_VibMode_Sta)  "<CAN2_IVI_SWC_VibMode_Sta>"
  IVISWCVibModeSta/1(VHAL_IVISWCVibModeSta_enum) -> VHAL_IVISWCVibModeSta_enum/1
  [DT_CAN2_SG_IVI1] -> bus_selector22/1
  bus_selector22/1 -> IVIStoppingUnlockSWSta/1(IVI_Stopping_Unlock_SW_Sta)  "<CAN2_IVI_Stopping_Unlock_SW_Sta>"
  IVIStoppingUnlockSWSta/1(VHAL_IVIStoppingUnlockSWSta_flg) -> VHAL_IVIStoppingUnlockSWSta_flg/1
  [DT_CAN2_SG_IVI1] -> bus_selector23/1
  bus_selector23/1 -> IVITimeCheck/1(IVI_Time_Check)  "<CAN2_IVI_Time_Check>"
  IVITimeCheck/1(VHAL_IVITimeCheck_enum) -> VHAL_IVITimeCheck_enum/1
  [DT_CAN2_SG_IVI1] -> bus_selector24/1
  bus_selector24/1 -> IVITimeDay/1(IVI_Time_Day)  "<CAN2_IVI_Time_Day>"
  IVITimeDay/1(VHAL_IVITimeDay_DAY) -> VHAL_IVITimeDay_DAY/1
  [DT_CAN2_SG_IVI1] -> bus_selector25/1
  bus_selector25/1 -> IVITimeHour/1(IVI_Time_Hour)  "<CAN2_IVI_Time_Hour>"
  IVITimeHour/1(VHAL_IVITimeHour_hr) -> VHAL_IVITimeHour_hr/1
  [DT_CAN2_SG_IVI1] -> bus_selector26/1
  bus_selector26/1 -> IVITimeMinute/1(IVI_Time_Minute)  "<CAN2_IVI_Time_Minute>"
  IVITimeMinute/1(VHAL_IVITimeMinute_min) -> VHAL_IVITimeMinute_min/1
  [DT_CAN2_SG_IVI1] -> bus_selector27/1
  bus_selector27/1 -> IVITimeMonth/1(IVI_Time_Month)  "<CAN2_IVI_Time_Month>"
  IVITimeMonth/1(VHAL_IVITimeMonth_MONTH) -> VHAL_IVITimeMonth_MONTH/1
  [DT_CAN2_SG_IVI1] -> bus_selector28/1
  bus_selector28/1 -> IVITimeSecond/1(IVI_Time_Second)  "<CAN2_IVI_Time_Second>"
  IVITimeSecond/1(VHAL_IVITimeSecond_s) -> VHAL_IVITimeSecond_s/1
  [DT_CAN2_SG_IVI1] -> bus_selector29/1
  bus_selector29/1 -> IVITimeYear/1(IVI_Time_Year)  "<CAN2_IVI_Time_Year>"
  IVITimeYear/1(VHAL_IVITimeYear_YEAR) -> VHAL_IVITimeYear_YEAR/1
  [DT_CAN2_SG_IVI1] -> bus_selector30/1
  bus_selector30/1 -> IVIWPTCSWSta/1(IVI_WPTC_SW_Sta)  "<CAN2_IVI_WPTC_SW_Sta>"
  IVIWPTCSWSta/1(VHAL_IVIWPTCSWSta_flg) -> VHAL_IVIWPTCSWSta_flg/1
  [DT_CAN2_SG_IVI1] -> bus_selector31/1
  bus_selector31/1 -> IVIsigScreenReqSta/1(IVI_sigScreenReq_Sta)  "<CAN2_IVI_sigScreenReq_Sta>"
  IVIsigScreenReqSta/1(VHAL_IVIsigScreenReqSta_flg) -> VHAL_IVIsigScreenReqSta_flg/1
  [DT_CAN2_SG_IVI1] -> bus_selector32/1
  bus_selector32/1 -> LINKtoDrive/1(LINKtoDrive)  "<CAN2_LINKtoDrive>"
  LINKtoDrive/1(VHAL_LINKtoDrive_flg) -> VHAL_LINKtoDrive_flg/1
  [DT_CAN2_SG_IVI1] -> bus_selector33/1
  bus_selector33/1 -> OpenDrOpenWdoSW/1(OpenDrOpenWdo_SW)  "<CAN2_OpenDrOpenWdo_SW>"
  OpenDrOpenWdoSW/1(VHAL_OpenDrOpenWdoSW_flg) -> VHAL_OpenDrOpenWdoSW_flg/1
  [DT_CAN2_SG_IVI1] -> bus_selector34/1
  bus_selector34/1 -> PWCONTINUEUSE/1(PW_CONTINUE_USE)  "<CAN2_PW_CONTINUE_USE>"
  PWCONTINUEUSE/1(VHAL_PWCONTINUEUSE_flg) -> VHAL_PWCONTINUEUSE_flg/1
  [DT_CAN2_SG_IVI1] -> bus_selector35/1
  bus_selector35/1 -> SmartEcoModeSW/1(SmartEco_Mode_SW)  "<CAN2_SmartEco_Mode_SW>"
  SmartEcoModeSW/1(VHAL_SmartEcoModeSW_flg) -> VHAL_SmartEcoModeSW_flg/1
  [DT_CAN2_SG_IVI1] -> bus_selector36/1
  bus_selector36/1 -> UserSet/1(UserSet)  "<CAN2_UserSet>"
  UserSet/1(VHAL_UserSet_enum) -> VHAL_UserSet_enum/1
